simulink model "display_data2"  (R2024a)
settings: Solver=VariableStepAuto  StartTime=0.0  StopTime=inf  RelTol=1e-3
libraries: ros2lib x6, sharedtransform x3, simulink_extras x3
settings Model: Creator=eswarm  LastModifiedBy=eswarm

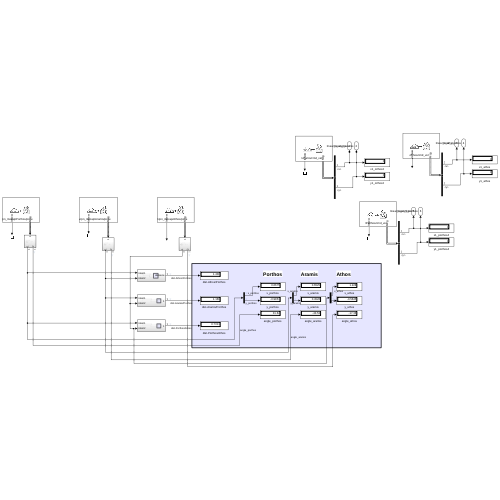
[thumbnail: Simulink's stored preview of the top-level diagram]
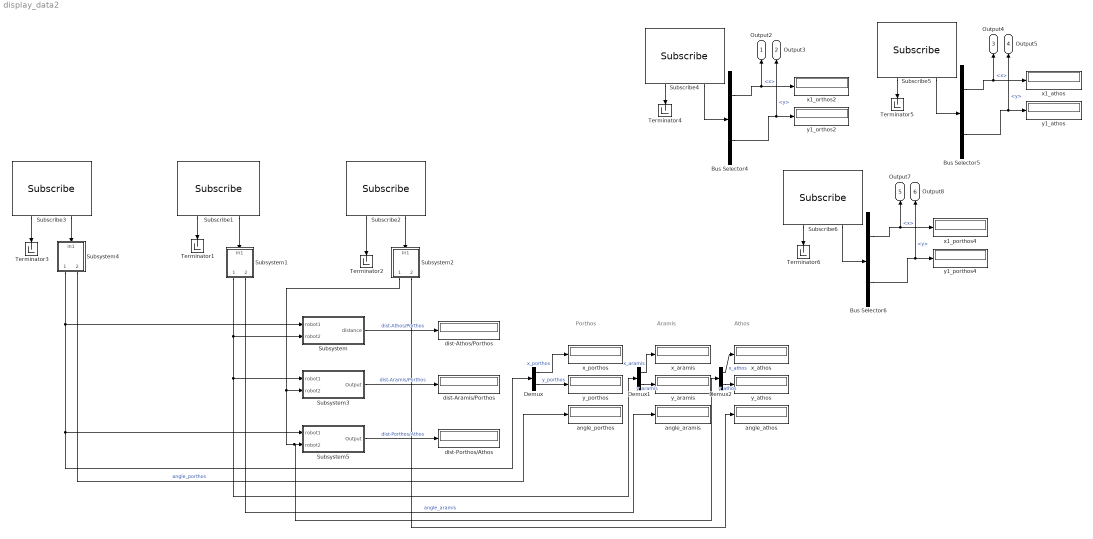
== system display_data2 ==
  note: Porthos
  note: Aramis
  note: Athos
  Bus Selector4 : BusSelector  OutputSignals=linear.x,linear.y
  Bus Selector5 : BusSelector  OutputSignals=linear.x,linear.y
  Bus Selector6 : BusSelector  OutputSignals=linear.x,linear.y
  Demux : Demux  Outputs=2
  Demux1 : Demux  Outputs=2
  Demux2 : Demux  Outputs=2
  Subscribe1 : ros2lib/Subscribe  topicSource=Select from ROS network  topic=/vrpn_mocap/Aramis/pose  messageType=geometry_msgs/PoseStamped  sampleTime=0.1  QOSHistory=Keep last  QOSDepth=1  QOSReliability=Best effort  QOSDurability=Volatile  QOSDeadline=Inf  QOSLifespan=Inf  QOSLiveliness=Automatic  QOSLeaseDuration=Inf  QOSAvoidROSNamespaceConventions=off
  Subscribe2 : ros2lib/Subscribe  topicSource=Select from ROS network  topic=/vrpn_mocap/Athos/pose  messageType=geometry_msgs/PoseStamped  sampleTime=0.1  QOSHistory=Keep last  QOSDepth=1  QOSReliability=Best effort  QOSDurability=Volatile  QOSDeadline=Inf  QOSLifespan=Inf  QOSLiveliness=Automatic  QOSLeaseDuration=Inf  QOSAvoidROSNamespaceConventions=off
  Subscribe3 : ros2lib/Subscribe  topicSource=Select from ROS network  topic=/vrpn_mocap/Porthos/pose  messageType=geometry_msgs/PoseStamped  sampleTime=0.1  QOSHistory=Keep last  QOSDepth=1  QOSReliability=Best effort  QOSDurability=Volatile  QOSDeadline=Inf  QOSLifespan=Inf  QOSLiveliness=Automatic  QOSLeaseDuration=Inf  QOSAvoidROSNamespaceConventions=off
  Subscribe4 : ros2lib/Subscribe  topicSource=Select from ROS network  topic=/Aramis/cmd_vel  messageType=geometry_msgs/Twist  sampleTime=0.1  QOSHistory=Keep last  QOSDepth=1  QOSReliability=Best effort  QOSDurability=Volatile  QOSDeadline=Inf  QOSLifespan=Inf  QOSLiveliness=Automatic  QOSLeaseDuration=Inf  QOSAvoidROSNamespaceConventions=off
  Subscribe5 : ros2lib/Subscribe  topicSource=Select from ROS network  topic=/Athos/cmd_vel  messageType=geometry_msgs/Twist  sampleTime=0.1  QOSHistory=Keep last  QOSDepth=1  QOSReliability=Best effort  QOSDurability=Volatile  QOSDeadline=Inf  QOSLifespan=Inf  QOSLiveliness=Automatic  QOSLeaseDuration=Inf  QOSAvoidROSNamespaceConventions=off
  Subscribe6 : ros2lib/Subscribe  topicSource=Select from ROS network  topic=/Porthos/cmd_vel  messageType=geometry_msgs/Twist  sampleTime=0.1  QOSHistory=Keep last  QOSDepth=1  QOSReliability=Best effort  QOSDurability=Volatile  QOSDeadline=Inf  QOSLifespan=Inf  QOSLiveliness=Automatic  QOSLeaseDuration=Inf  QOSAvoidROSNamespaceConventions=off
  Subsystem : Subsystem
  Subsystem1 : Subsystem
  Subsystem2 : Subsystem
  Subsystem3 : Subsystem
  Subsystem4 : Subsystem
  Subsystem5 : Subsystem
  Terminator{1..6} (6 alike) : Terminator
  angle_aramis : Display
  angle_athos : Display
  angle_porthos : Display
  dist-Aramis/Porthos : Display
  dist-Athos/Porthos : Display
  dist-Porthos/Athos : Display
  x1_athos : Display
  x1_orthos2 : Display
  x1_porthos4 : Display
  x_aramis : Display
  x_athos : Display
  x_porthos : Display
  y1_athos : Display
  y1_orthos2 : Display
  y1_porthos4 : Display
  y_aramis : Display
  y_athos : Display
  y_porthos : Display
  Output2 : Outport  SignalName=linear_x_aramis
  Output3 : Outport  Port=2  SignalName=linear_y_aramis
  Output4 : Outport  Port=3  SignalName=linear_x_athos
  Output5 : Outport  Port=4  SignalName=linear_y_athos
  Output7 : Outport  Port=5  SignalName=linear_x_porthos
  Output8 : Outport  Port=6  SignalName=linear_y_porthos
  wires:
  Bus Selector5/2 -> Output5/1, y1_athos/1  "<y>"
  Subscribe5/1 -> Terminator5/1
  Subscribe1/1 -> Terminator1/1
  Bus Selector5/1 -> Output4/1, x1_athos/1  "<x>"
  Subscribe5/2 -> Bus Selector5/1
  Bus Selector4/2 -> Output3/1, y1_orthos2/1  "<y>"
  Subscribe4/1 -> Terminator4/1
  Bus Selector4/1 -> Output2/1, x1_orthos2/1  "<x>"
  Subscribe2/1 -> Terminator2/1
  Subscribe4/2 -> Bus Selector4/1
  Subscribe3/1 -> Terminator3/1
  Subscribe3/2 -> Subsystem4/1(In1)
  Subscribe6/1 -> Terminator6/1
  Bus Selector6/1 -> Output7/1, x1_porthos4/1  "<x>"
  Subscribe6/2 -> Bus Selector6/1
  Bus Selector6/2 -> Output8/1, y1_porthos4/1  "<y>"
  Subscribe1/2 -> Subsystem1/1(In1)
  Subscribe2/2 -> Subsystem2/1(In1)
  Subsystem4/1(Output11) -> Subsystem5/1(robot1), Demux/1, Subsystem/1(robot1)
  Subsystem1/1(Output11) -> Subsystem3/1(robot1), Demux1/1, Subsystem/2(robot2)
  Subsystem2/1(Output11) -> Subsystem3/2(robot2), Subsystem5/2(robot2), Demux2/1
  Subsystem3/1(Output) -> dist-Aramis/Porthos/1  "dist-Aramis/Porthos"
  Subsystem5/1(Output) -> dist-Porthos/Athos/1  "dist-Porthos/Athos"
  Demux/1 -> x_porthos/1  "x_porthos"
  Demux/2 -> y_porthos/1  "y_porthos"
  Subsystem4/2(Out1) -> angle_porthos/1  "angle_porthos"
  Demux1/1 -> x_aramis/1  "x_aramis"
  Demux1/2 -> y_aramis/1  "y_aramis"
  Subsystem1/2(Out1) -> angle_aramis/1  "angle_aramis"
  Demux2/2 -> y_athos/1  "y_athos"
  Demux2/1 -> x_athos/1  "x_athos"
  Subsystem2/2(Out1) -> angle_athos/1
  Subsystem/1(distance) -> dist-Athos/Porthos/1  "dist-Athos/Porthos"

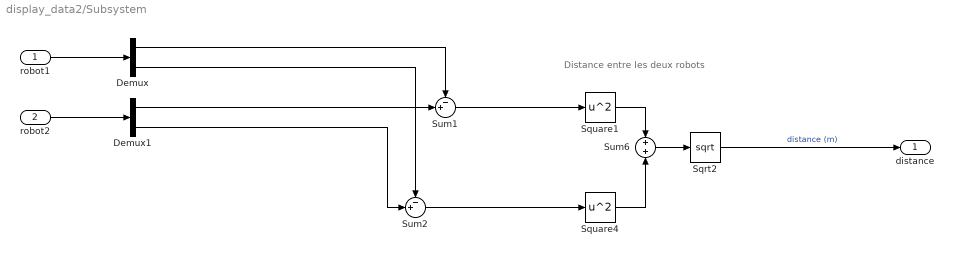
== system display_data2/Subsystem ==
  note: Distance entre les deux robots
  robot1 : Inport
  robot2 : Inport  Port=2
  Demux : Demux  Outputs=2
  Demux1 : Demux  Outputs=2
  Sqrt2 : Sqrt
  Square1 : Math  Operator=square
  Square4 : Math  Operator=square
  Sum1 : Sum  Inputs=-+|
  Sum2 : Sum  Inputs=-+|
  Sum6 : Sum  Inputs=+|+
  distance : Outport
  wires:
  Demux1/2 -> Sum2/2
  Square1/1 -> Sum6/1
  Sum2/1 -> Square4/1
  Sum1/1 -> Square1/1
  Sum6/1 -> Sqrt2/1
  Demux/2 -> Sum2/1
  Square4/1 -> Sum6/2
  Demux/1 -> Sum1/1
  Sqrt2/1 -> distance/1  "distance (m)"
  robot1/1 -> Demux/1
  robot2/1 -> Demux1/1
  Demux1/1 -> Sum1/2

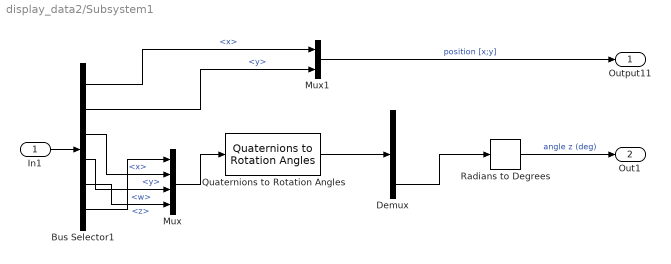
== system display_data2/Subsystem1 ==
  In1 : Inport
  Bus Selector1 : BusSelector  OutputSignals=pose.position.x,pose.position.y,pose.orientation.x,pose.orientation.y,pose.orientation.z,pose.orientation.w
  Demux : Demux  Outputs=3
  Mux : Mux
  Mux1 : Mux  Inputs=2
  Quaternions to Rotation Angles : sharedtransform/Quaternions to Rotation Angles  rotationOrder=XYZ  aMode=aMode
  Radians to Degrees : simulink_extras/Transformations/Radians to Degrees
  Output11 : Outport
  Out1 : Outport  Port=2
  wires:
  Quaternions to Rotation Angles/1 -> Demux/1
  Radians to Degrees/1 -> Out1/1  "angle z (deg)"
  Demux/3 -> Radians to Degrees/1
  In1/1 -> Bus Selector1/1
  Mux/1 -> Quaternions to Rotation Angles/1
  Bus Selector1/6 -> Mux/1  "<w>"
  Bus Selector1/3 -> Mux/2  "<x>"
  Bus Selector1/4 -> Mux/3  "<y>"
  Bus Selector1/5 -> Mux/4  "<z>"
  Bus Selector1/2 -> Mux1/2  "<y>"
  Bus Selector1/1 -> Mux1/1  "<x>"
  Mux1/1 -> Output11/1  "position [x;y]"

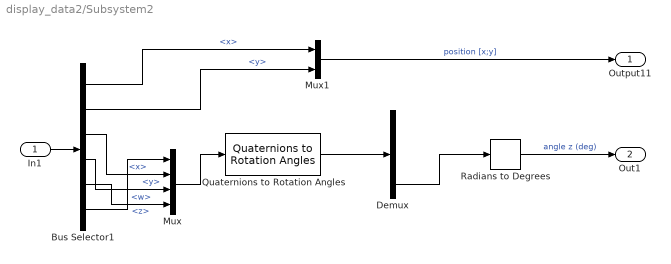
== system display_data2/Subsystem2 ==
  In1 : Inport
  Bus Selector1 : BusSelector  OutputSignals=pose.position.x,pose.position.y,pose.orientation.x,pose.orientation.y,pose.orientation.z,pose.orientation.w
  Demux : Demux  Outputs=3
  Mux : Mux
  Mux1 : Mux  Inputs=2
  Quaternions to Rotation Angles : sharedtransform/Quaternions to Rotation Angles  rotationOrder=XYZ  aMode=aMode
  Radians to Degrees : simulink_extras/Transformations/Radians to Degrees
  Output11 : Outport
  Out1 : Outport  Port=2
  wires:
  Quaternions to Rotation Angles/1 -> Demux/1
  Radians to Degrees/1 -> Out1/1  "angle z (deg)"
  Demux/3 -> Radians to Degrees/1
  In1/1 -> Bus Selector1/1
  Mux/1 -> Quaternions to Rotation Angles/1
  Bus Selector1/6 -> Mux/1  "<w>"
  Bus Selector1/3 -> Mux/2  "<x>"
  Bus Selector1/4 -> Mux/3  "<y>"
  Bus Selector1/5 -> Mux/4  "<z>"
  Bus Selector1/2 -> Mux1/2  "<y>"
  Bus Selector1/1 -> Mux1/1  "<x>"
  Mux1/1 -> Output11/1  "position [x;y]"

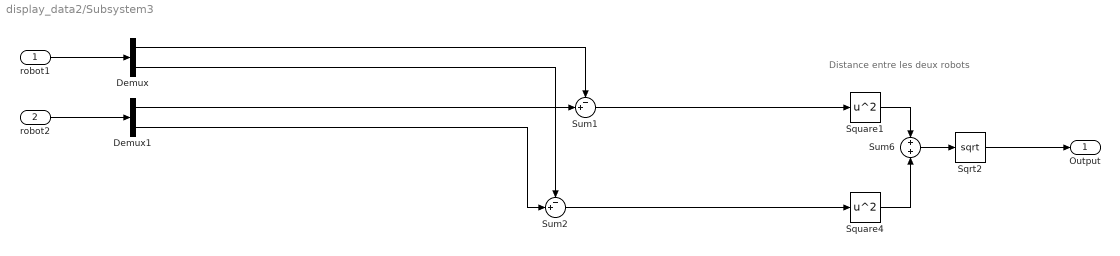
== system display_data2/Subsystem3 ==
  note: Distance entre les deux robots
  robot1 : Inport
  robot2 : Inport  Port=2
  Demux : Demux  Outputs=2
  Demux1 : Demux  Outputs=2
  Sqrt2 : Sqrt
  Square1 : Math  Operator=square
  Square4 : Math  Operator=square
  Sum1 : Sum  Inputs=-+|
  Sum2 : Sum  Inputs=-+|
  Sum6 : Sum  Inputs=+|+
  Output : Outport
  wires:
  Demux1/2 -> Sum2/2
  Square1/1 -> Sum6/1
  Sum2/1 -> Square4/1
  Sum1/1 -> Square1/1
  Sum6/1 -> Sqrt2/1
  Demux/2 -> Sum2/1
  Square4/1 -> Sum6/2
  Demux/1 -> Sum1/1
  Sqrt2/1 -> Output/1
  robot1/1 -> Demux/1
  robot2/1 -> Demux1/1
  Demux1/1 -> Sum1/2

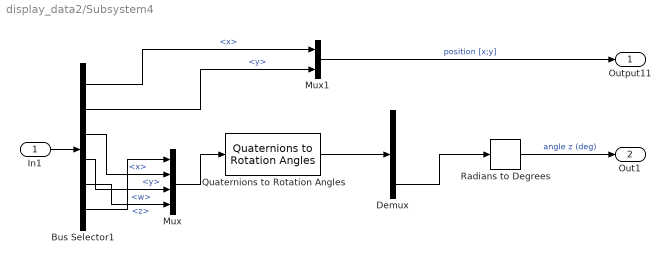
== system display_data2/Subsystem4 ==
  In1 : Inport
  Bus Selector1 : BusSelector  OutputSignals=pose.position.x,pose.position.y,pose.orientation.x,pose.orientation.y,pose.orientation.z,pose.orientation.w
  Demux : Demux  Outputs=3
  Mux : Mux
  Mux1 : Mux  Inputs=2
  Quaternions to Rotation Angles : sharedtransform/Quaternions to Rotation Angles  rotationOrder=XYZ  aMode=aMode
  Radians to Degrees : simulink_extras/Transformations/Radians to Degrees
  Output11 : Outport
  Out1 : Outport  Port=2
  wires:
  Quaternions to Rotation Angles/1 -> Demux/1
  Radians to Degrees/1 -> Out1/1  "angle z (deg)"
  Demux/3 -> Radians to Degrees/1
  In1/1 -> Bus Selector1/1
  Mux/1 -> Quaternions to Rotation Angles/1
  Bus Selector1/6 -> Mux/1  "<w>"
  Bus Selector1/3 -> Mux/2  "<x>"
  Bus Selector1/4 -> Mux/3  "<y>"
  Bus Selector1/5 -> Mux/4  "<z>"
  Bus Selector1/2 -> Mux1/2  "<y>"
  Bus Selector1/1 -> Mux1/1  "<x>"
  Mux1/1 -> Output11/1  "position [x;y]"

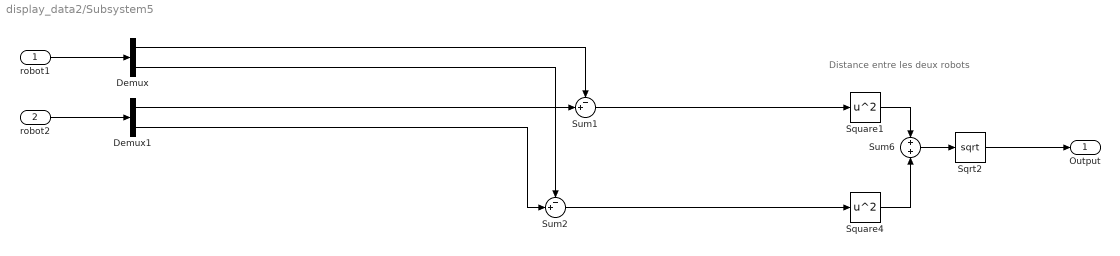
== system display_data2/Subsystem5 ==
  note: Distance entre les deux robots
  robot1 : Inport
  robot2 : Inport  Port=2
  Demux : Demux  Outputs=2
  Demux1 : Demux  Outputs=2
  Sqrt2 : Sqrt
  Square1 : Math  Operator=square
  Square4 : Math  Operator=square
  Sum1 : Sum  Inputs=-+|
  Sum2 : Sum  Inputs=-+|
  Sum6 : Sum  Inputs=+|+
  Output : Outport
  wires:
  Demux1/2 -> Sum2/2
  Square1/1 -> Sum6/1
  Sum2/1 -> Square4/1
  Sum1/1 -> Square1/1
  Sum6/1 -> Sqrt2/1
  Demux/2 -> Sum2/1
  Square4/1 -> Sum6/2
  Demux/1 -> Sum1/1
  Sqrt2/1 -> Output/1
  robot1/1 -> Demux/1
  robot2/1 -> Demux1/1
  Demux1/1 -> Sum1/2
